simulink model "ESC_sim"  (R2021b)
settings: Solver=ode1  StartTime=0.0  StopTime=5  FixedStep=0.001  RelTol=1e-3
values from neighbouring files (symbols this model uses):
  LT_in_Delta_big = [0 0.00436332312999 0.00872664625997 0.01308996939 0.0174532925199 0.0218166156499 0.0261799387799 0.0305432619099 0.0349065850399 0.0392699081699 0.0436332312999 0.0479965544298 ... (81 elements, 1x81)]    [LT_big_ramp.mat]
  LT_in_Vx_big = [5 5.5 6 6.5 7 7.5 8 8.5 9 9.5 10 10.5 ... (111 elements, 1x111)]    [LT_big_ramp.mat]
  LT_YawRate_big = [0 0 0 0 0 0 0 0 0 0 0 0 ... (8991 elements, 111x81)]    [LT_big_ramp.mat]
undefined symbols (not defined in the file or in its folder): car
libraries: car_library x2, slpidlib x1
settings Model: Creator=efrem  LastModifiedBy=uzakotim

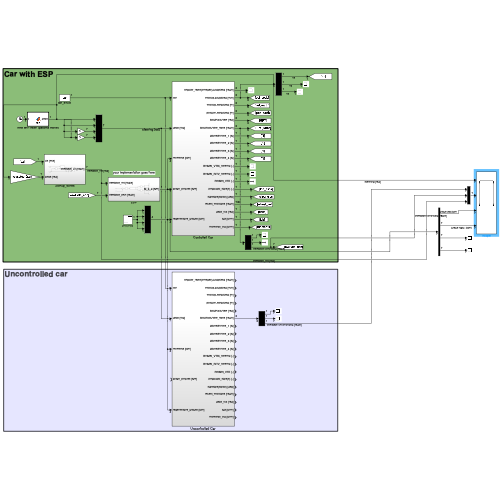
[thumbnail: Simulink's stored preview of the top-level diagram]
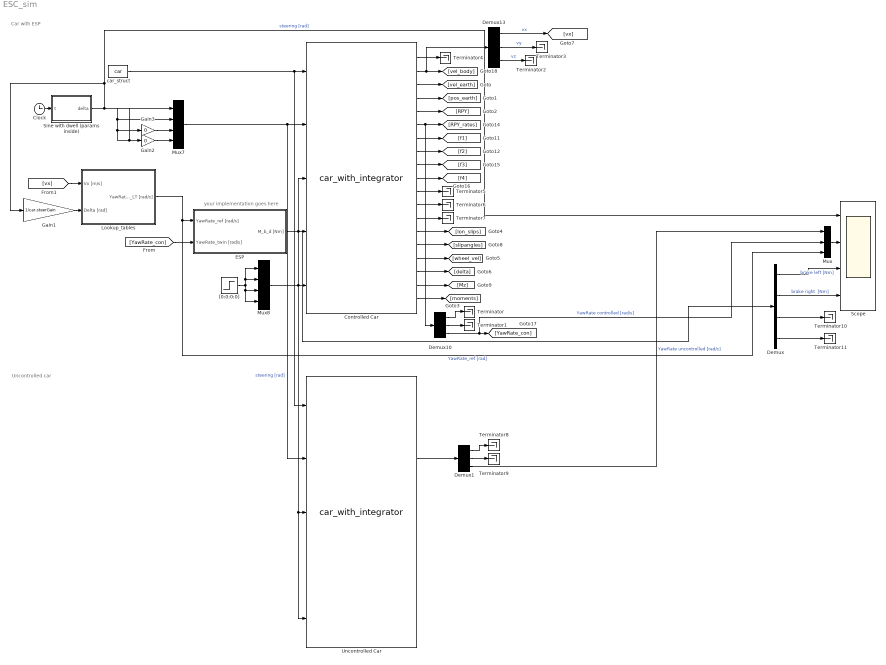
== system ESC_sim ==
  note: your implementation goes here
  note: Uncontrolled car
  note: Car with ESP
  Clock : Clock
  Controlled Car : car_library/car_with_integrator  SystemSampleTime=-1  VariantActivationTime=update diagram  Latency=0  AutoFrameSizeCalculation=off
  Demux : Demux
  Demux1 : Demux  Outputs=3
  Demux10 : Demux  Outputs=3
  Demux13 : Demux  Outputs=3
  ESP : Subsystem
  Gain1 : Gain  Gain=1/car.steerGain
  Gain2 : Gain  Gain=0
  Gain3 : Gain  Gain=0
  Lookup_tables : Subsystem
  Mux : Mux  Inputs=3
  Mux7 : Mux
  Mux8 : Mux
  Scope : Scope  NumInputPorts=4
  Sine with dwell (params inside) : MATLAB Function  TreatAsAtomicUnit=on
  Terminator{,1..11} (12 alike) : Terminator
  Uncontrolled Car : car_library/car_with_integrator  SystemSampleTime=-1  VariantActivationTime=update diagram  Latency=0  AutoFrameSizeCalculation=off
  "[0;0;0;0]" : Step  Time=0  After=0  SampleTime=0
  car_struct : Constant  Value=car  OutDataTypeStr=Bus: car_bus
  wires:
  Controlled Car/11 -> Terminator5/1
  ESP/1(M_b_d [Nm]) -> Demux/1, Controlled Car/4
  Controlled Car/13 -> Terminator7/1
  Sine with dwell (params inside)/1(delta) -> Scope/1, Gain1/1, Mux7/1, Mux7/2, Gain3/1, Gain2/1  "steering [rad]"
  Controlled Car/17 -> [delta]
  Controlled Car/15 -> [slipangles]
  Controlled Car/19 -> [moments]
  Controlled Car/16 -> [wheel_vel]
  Controlled Car/5 -> [RPY]
  Controlled Car/1 -> Terminator4/1
  Gain3/1 -> Mux7/3
  Mux8/1 -> Uncontrolled Car/3, Uncontrolled Car/5, Controlled Car/3, Controlled Car/5
  Controlled Car/18 -> [Mz]
  Controlled Car/7 -> [f1]
  Demux10/3 -> Mux/2, [YawRate_con]  "YawRate controlled [rad/s]"
  Controlled Car/6 -> [RPY_rates], Demux10/1
  Gain2/1 -> Mux7/4
  "[0;0;0;0]"/1 -> Mux8/2, Mux8/1, Mux8/4, Mux8/3
  car_struct/1 -> Uncontrolled Car/1, Controlled Car/1
  Controlled Car/4 -> [pos_earth]
  Controlled Car/3 -> [vel_earth]
  Controlled Car/8 -> [f2]
  Mux7/1 -> Uncontrolled Car/2, Controlled Car/2  "steering [rad]"
  Demux10/1 -> Terminator/1
  Controlled Car/10 -> [f4]
  Controlled Car/9 -> [f3]
  Controlled Car/12 -> Terminator6/1
  Demux10/2 -> Terminator1/1
  Controlled Car/14 -> [lon_slips]
  Controlled Car/2 -> Demux13/1, [vel_body]
  Clock/1 -> Sine with dwell (params inside)/1(t)
  [YawRate_con] -> ESP/2(YawRate_twin [rad/s])
  Demux13/2 -> Terminator3/1  "vy"
  Demux13/1 -> [vx]  "vx"
  Demux13/3 -> Terminator2/1  "vz"
  [vx] -> Lookup_tables/1(Vx [m/s])
  Lookup_tables/1(YawRate_LT [rad/s]) -> Mux/3, ESP/1(YawRate_ref [rad/s])  "YawRate_ref [rad]"
  Demux1/1 -> Terminator8/1
  Demux1/2 -> Terminator9/1
  Uncontrolled Car/6 -> Demux1/1
  Demux1/3 -> Mux/1  "YawRate uncontrolled [rad/s]"
  Demux/1 -> Scope/3  "brake left [Nm]"
  Demux/2 -> Scope/4  "brake right  [Nm]"
  Demux/3 -> Terminator10/1
  Demux/4 -> Terminator11/1
  Gain1/1 -> Lookup_tables/2(Delta [rad])
  Mux/1 -> Scope/2

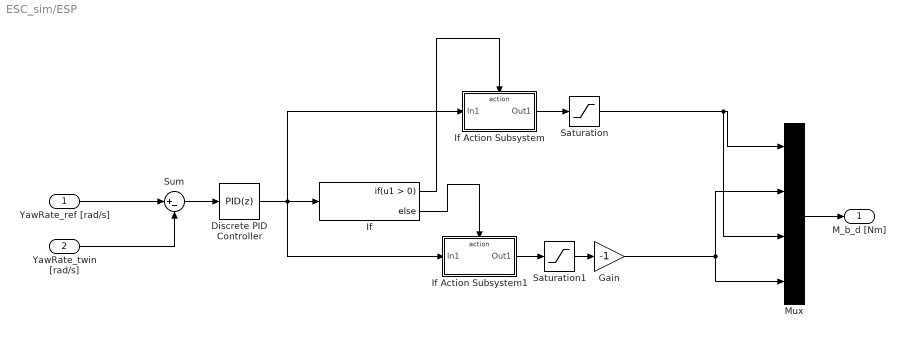
== system ESC_sim/ESP ==
  YawRate_ref [rad/s] : Inport
  YawRate_twin [rad/s] : Inport  Port=2
  Discrete PID Controller : slpidlib/PID Controller  Controller=PID  Form=Parallel  TimeDomain=Discrete-time  UseExternalTs=off  SampleTime=-1  IntegratorMethod=Forward Euler  FilterMethod=Forward Euler  ControllerParametersSource=internal  P=8750  I=0  D=100  UseFilter=on  N=100  TunerSelectOption=Transfer Function Based (PID Tuner App)  InitialConditionSource=internal  InitialConditionForIntegrator=0  InitialConditionForFilter=0  DifferentiatorICPrevScaledInput=0  ExternalReset=none  TrackingMode=off  Kt=1  LimitOutput=off  SatLimitsSource=internal  UpperSaturationLimit=inf  LowerSaturationLimit=-inf  LinearizeAsGain=off  AntiWindupMode=none  Kb=1  POutMin=[]  POutMax=[]  IOutMin=[]  IOutMax=[]  DOutMin=[]  DOutMax=[]  NOutMin=[]  NOutMax=[]  SumOutMin=[]  SumOutMax=[]  SaturationOutMin=[]  SaturationOutMax=[]  PParamMin=[]  PParamMax=[]  IParamMin=[]  IParamMax=[]  DParamMin=[]  DParamMax=[]  NParamMin=[]  NParamMax=[]  KbParamMin=[]  KbParamMax=[]  KtParamMin=[]  KtParamMax=[]  KbOutMin=[]  KbOutMax=[]  KtOutMin=[]  KtOutMax=[]  IntegratorOutMin=[]  IntegratorOutMax=[]  FilterOutMin=[]  FilterOutMax=[]  SumI1OutMin=[]  SumI1OutMax=[]  SumI2OutMin=[]  SumI2OutMax=[]  SumI3OutMin=[]  SumI3OutMax=[]  SumI4OutMin=[]  SumI4OutMax=[]  SumDOutMin=[]  SumDOutMax=[]  DifferentiatorOutMin=[]  DifferentiatorOutMax=[]  FilterDiffOutCoefMin=[]  FilterDiffOutCoefMax=[]  ReciprocalOutMin=[]  ReciprocalOutMax=[]  SumDenOutMin=[]  SumDenOutMax=[]  SumNumOutMin=[]  SumNumOutMax=[]  DivideOutMin=[]  DivideOutMax=[]  UdiffTsProdOutMin=[]  UdiffTsProdOutMax=[]  NTsProdOutMin=[]  NTsProdOutMax=[]  UintegralTsProdOutMin=[]  UintegralTsProdOutMax=[]  UngainTsProdOutMin=[]  UngainTsProdOutMax=[]  IntegratorContinuousStateAttributes=''  IntegratorStateMustResolveToSignalObject=off  IntegratorRTWStateStorageClass=Auto  FilterContinuousStateAttributes=''  FilterStateMustResolveToSignalObject=off  FilterRTWStateStorageClass=Auto  ParallelPVariant=InternalParameters  IdealPVariant=Disabled  IVariant=InternalParameters  DVariant=InternalParameters  IntegratorVariant=Discrete  SatVariant=Disabled  AWVariant=Passthrough  PCopyVariant=Disabled  TRVariant=Disabled  FdbkBlocksVariant=Forward  IdealPFdbkVariant=Disabled  SatFdbkVariant=Disabled  DerivativeFilterVariant=ForwardEulerFilter  NVariant=InternalParameters  NCopyVariant=Disabled  FilterICVariant=InternalICsFilter  IntegratorICVariant=InternalICs  ExternalResetVariant=Disabled  TRSumVariant=Passthrough  SumFdbkVariant=Disabled  SumVariant=Sum_PID  TsampFilterVariant=InternalTs  TsampNgainVariant=Passthrough  TsampIntegralVariant=Passthrough  ExternalSaturationOutDataTypeStr=Inherit: Same as second input
  Gain : Gain  Gain=-1
  If : If
  If Action Subsystem : Subsystem  TreatAsAtomicUnit=on
  If Action Subsystem1 : Subsystem  TreatAsAtomicUnit=on
  Mux : Mux
  Saturation : Saturate  UpperLimit=2000  LowerLimit=0
  Saturation1 : Saturate  UpperLimit=0  LowerLimit=-2000
  Sum : Sum  Inputs=|+-
  M_b_d [Nm] : Outport
  wires:
  Mux/1 -> M_b_d [Nm]/1
  YawRate_ref [rad/s]/1 -> Sum/1
  YawRate_twin [rad/s]/1 -> Sum/2
  Sum/1 -> Discrete PID Controller/1
  If Action Subsystem/1(Out1) -> Saturation/1
  If Action Subsystem1/1(Out1) -> Saturation1/1
  Discrete PID Controller/1 -> If Action Subsystem/1(In1), If/1, If Action Subsystem1/1(In1)
  If/1 -> If Action Subsystem/Action
  If/2 -> If Action Subsystem1/Action
  Saturation1/1 -> Gain/1
  Saturation/1 -> Mux/3, Mux/1
  Gain/1 -> Mux/2, Mux/4

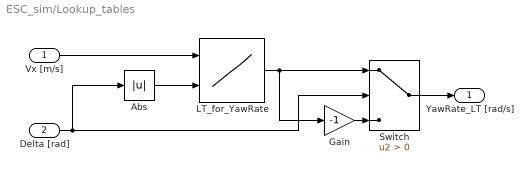
== system ESC_sim/Lookup_tables ==
  Vx [m/s] : Inport
  Delta [rad] : Inport  Port=2
  Abs : Abs
  Gain : Gain  Gain=-1
  LT_for_YawRate : Lookup_n-D  BreakpointsForDimension1=LT_in_Vx_big  BreakpointsForDimension2=LT_in_Delta_big  Table=LT_YawRate_big  InternalRulePriority=Speed  RndMeth=Simplest  InputSameDT=on
      settings: InputPortMap=u0,u1
  Switch : Switch  Criteria=u2 > Threshold
  YawRate_LT [rad/s] : Outport
  wires:
  Delta [rad]/1 -> Switch/2, Abs/1
  Vx [m/s]/1 -> LT_for_YawRate/1
  LT_for_YawRate/1 -> Gain/1, Switch/1
  Abs/1 -> LT_for_YawRate/2
  Gain/1 -> Switch/3
  Switch/1 -> YawRate_LT [rad/s]/1

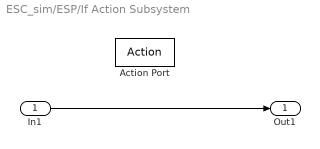
== system ESC_sim/ESP/If Action Subsystem ==
  In1 : Inport
  Action Port : ActionPort  ActionPortLabel=if(u1 > 0)
  Out1 : Outport
  wires:
  In1/1 -> Out1/1

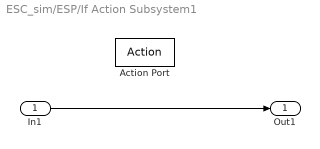
== system ESC_sim/ESP/If Action Subsystem1 ==
  In1 : Inport
  Action Port : ActionPort  ActionPortLabel=else
  Out1 : Outport
  wires:
  In1/1 -> Out1/1

== matlab function ESC_sim/Sine with dwell (params inside) ==
  data: t input; delta output
function delta = fcn(t)

% setting params
start_time = 0; % sec
time_of_maneuver = 2; % sec
time_of_dwell = 0.5; % sec
amplitude = 0.5; % rad

time_of_sinus = time_of_maneuver - time_of_dwell;
% time_of_dwell_start = 2*pi*(t-start_time)/time_of_sinus

delta = 0;

if t > start_time && t <= start_time + 0.75*time_of_sinus
    delta = amplitude*sin(2*pi*(t-start_time)/time_of_sinus);
end

if t > start_time + 0.75*time_of_sinus && t <= start_time + 0.75*time_of_sinus + time_of_dwell
    delta = -amplitude;
end

if t > start_time + 0.75*time_of_sinus + time_of_dwell && t <= start_time + time_of_maneuver
    delta = amplitude*sin(2*pi*(t-start_time-time_of_dwell)/time_of_sinus);
end
